simulink model "lin_att_model"  (R2024b)
settings: Solver=ode4  StartTime=0.0  StopTime=10  FixedStep=ST  RelTol=1e-3
values from neighbouring files (symbols this model uses):
  att_sp = 0    [FEL_RBFNN.m]    (also in results.m)
  B = [ 1/Ixx*lz_mr*T_mr_trim,          0,                 0 ... (first row only)    [parameters.m]
  B_inv = inv(B*B_dim)    [parameters.m]
  eta = 1    [FEL_RBFNN.m]
  f = [ 0; 0; Q_mr_trim/Izz]    [parameters.m]
  k = diag([3.7,5,10])    [FEL_RBFNN.m]
  lambda = diag([0.08,0.05,1.5])    [FEL_RBFNN.m]
  lat_cyc_range = [ -15 15 ]    [parameters.m]
  lon_cyc_range = [ -15 15 ]    [parameters.m]
  mr_coll_range = [ 7.5 25 ]    [parameters.m]
  NN_state = 1    [FEL_RBFNN.m]    (also in results.m)
  pilot_trim = [-0.11603144404 0.198191531149 -0.14266835704 0.401015389998]    [hover_trim.mat]
  sigma = linspace(1.2,4.2,neurons)'    [FEL_RBFNN.m]
  ST = 0.01    [parameters.m]
  T_flap = 16/GAMMA/OMEGA    (= 0.0932876459059)    [parameters.m]
  tr_coll_range = [ -20 20 ]    [parameters.m]
  W0 = zeros(neurons,3)    [FEL_RBFNN.m]
  x0 = linspace(-1,1,neurons)'    [FEL_RBFNN.m]
settings Model: Creator=fra62  LastModifiedBy=fra62

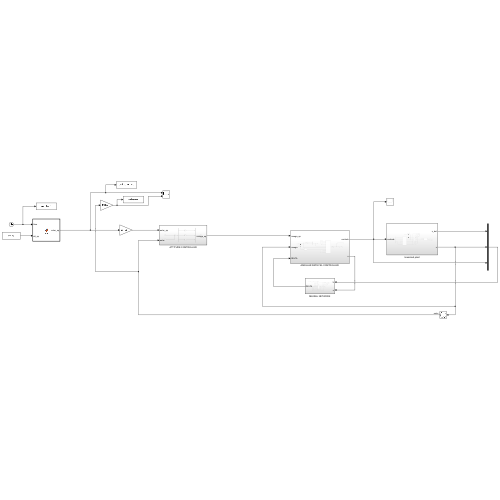
[thumbnail: Simulink's stored preview of the top-level diagram]
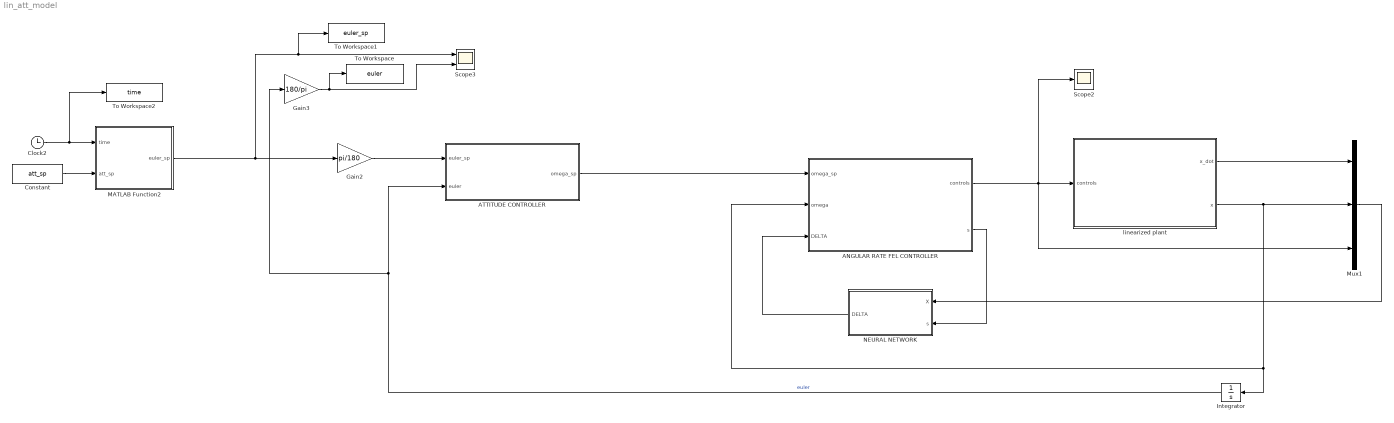
== system lin_att_model ==
  "ANGULAR RATE FEL CONTROLLER " : Subsystem
  ATTITUDE CONTROLLER : Subsystem
  Clock2 : Clock
  Constant : Constant  Value=att_sp
  Gain2 : Gain  Gain=pi/180
  Gain3 : Gain  Gain=180/pi
  Integrator : Integrator  WrapState=on
  MATLAB Function2 : MATLAB Function  TreatAsAtomicUnit=on
  Mux1 : Mux  Inputs=3
  "NEURAL NETWORK " : Subsystem
  Scope2 : Scope
  Scope3 : Scope  NumInputPorts=2
  To Workspace : ToWorkspace  VariableName=euler  SampleTime=-1
  To Workspace1 : ToWorkspace  VariableName=euler_sp  SampleTime=-1
  To Workspace2 : ToWorkspace  VariableName=time  SampleTime=-1
  linearized plant : Subsystem
  wires:
  "ANGULAR RATE FEL CONTROLLER "/1(controls) -> Scope2/1, linearized plant/1(controls), Mux1/3
  MATLAB Function2/1(euler_sp) -> Gain2/1, To Workspace1/1, Scope3/1
  Gain3/1 -> To Workspace/1, Scope3/2
  Clock2/1 -> To Workspace2/1, MATLAB Function2/1(time)
  linearized plant/2(x) -> Mux1/2, Integrator/1, "ANGULAR RATE FEL CONTROLLER "/2(omega)
  Mux1/1 -> "NEURAL NETWORK "/1(X)
  linearized plant/1(x_dot) -> Mux1/1
  "ANGULAR RATE FEL CONTROLLER "/2(s) -> "NEURAL NETWORK "/2(s)
  "NEURAL NETWORK "/1(DELTA) -> "ANGULAR RATE FEL CONTROLLER "/3(DELTA)
  Gain2/1 -> ATTITUDE CONTROLLER/1(euler_sp)
  Integrator/1 -> Gain3/1, ATTITUDE CONTROLLER/2(euler)  "euler"
  ATTITUDE CONTROLLER/1(omega_sp) -> "ANGULAR RATE FEL CONTROLLER "/1(omega_sp)
  Constant/1 -> MATLAB Function2/2(att_sp)

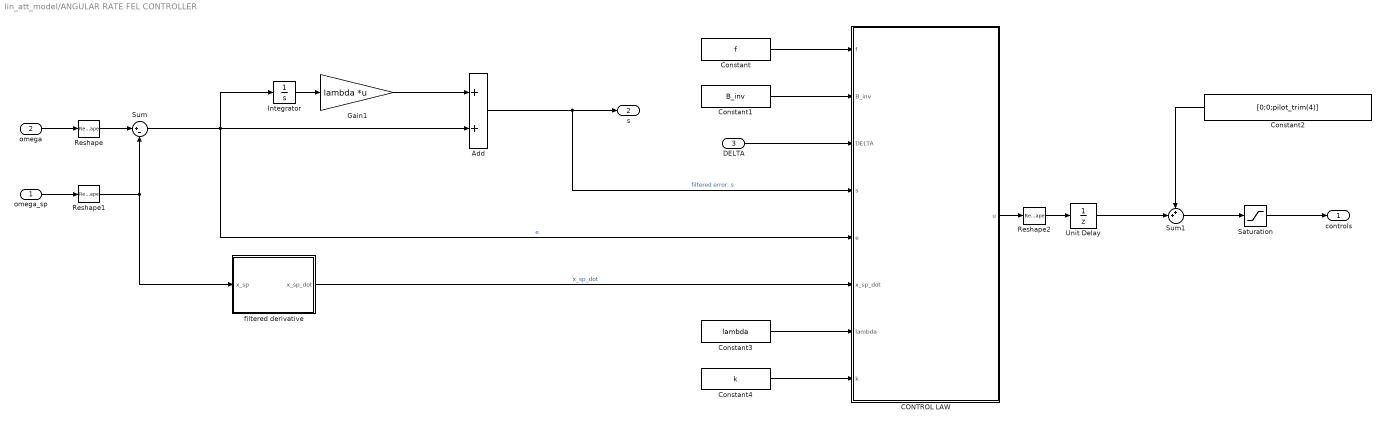
== system lin_att_model/ANGULAR RATE FEL CONTROLLER  ==
  omega_sp : Inport
  omega : Inport  Port=2
  DELTA : Inport  Port=3
  Add : Sum
  CONTROL LAW : MATLAB Function  TreatAsAtomicUnit=on
  Constant : Constant  Value=f
  Constant1 : Constant  Value=B_inv
  Constant2 : Constant  Value=[0;0;pilot_trim(4)]
  Constant3 : Constant  Value=lambda
  Constant4 : Constant  Value=k
  Gain1 : Gain  Gain=lambda  Multiplication=Matrix(K*u) (u vector)
  Integrator : Integrator
  Reshape : Reshape  OutputDimensionality=Column vector (2-D)
  Reshape1 : Reshape  OutputDimensionality=Column vector (2-D)
  Reshape2 : Reshape  OutputDimensionality=Column vector (2-D)
  Saturation : Saturate  UpperLimit=1  LowerLimit=-1
  Sum : Sum  Inputs=|+-
  Sum1 : Sum  Inputs=++|
  Unit Delay : UnitDelay  SampleTime=-1  HasFrameUpgradeWarning=on
  filtered derivative : Subsystem
  controls : Outport
  s : Outport  Port=2
  wires:
  CONTROL LAW/1(u) -> Reshape2/1
  Saturation/1 -> controls/1
  Constant/1 -> CONTROL LAW/1(f)
  Constant1/1 -> CONTROL LAW/2(B_inv)
  DELTA/1 -> CONTROL LAW/3(DELTA)
  Constant3/1 -> CONTROL LAW/7(lambda)
  Constant4/1 -> CONTROL LAW/8(k)
  omega_sp/1 -> Reshape1/1
  omega/1 -> Reshape/1
  Reshape1/1 -> filtered derivative/1(x_sp), Sum/2
  filtered derivative/1(x_sp_dot) -> CONTROL LAW/6(x_sp_dot)  "x_sp_dot"
  Sum/1 -> Integrator/1, Add/2, CONTROL LAW/5(e)  "e"
  Add/1 -> s/1, CONTROL LAW/4(s)  "filtered error: s"
  Gain1/1 -> Add/1
  Integrator/1 -> Gain1/1
  Reshape/1 -> Sum/1
  Reshape2/1 -> Unit Delay/1
  Unit Delay/1 -> Sum1/2
  Sum1/1 -> Saturation/1
  Constant2/1 -> Sum1/1

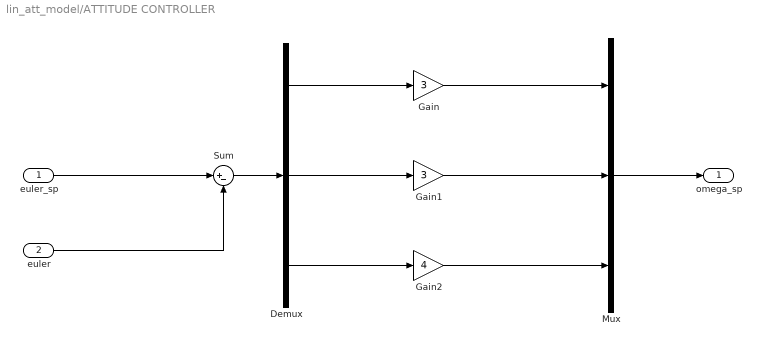
== system lin_att_model/ATTITUDE CONTROLLER ==
  euler_sp : Inport
  euler : Inport  Port=2
  Demux : Demux  Outputs=3
  Gain : Gain  Gain=3
  Gain1 : Gain  Gain=3
  Gain2 : Gain  Gain=4
  Mux : Mux  Inputs=3
  Sum : Sum  Inputs=|+-
  omega_sp : Outport
  wires:
  Gain2/1 -> Mux/3
  euler/1 -> Sum/2
  Mux/1 -> omega_sp/1
  Demux/3 -> Gain2/1
  Demux/2 -> Gain1/1
  Gain/1 -> Mux/1
  euler_sp/1 -> Sum/1
  Demux/1 -> Gain/1
  Sum/1 -> Demux/1
  Gain1/1 -> Mux/2

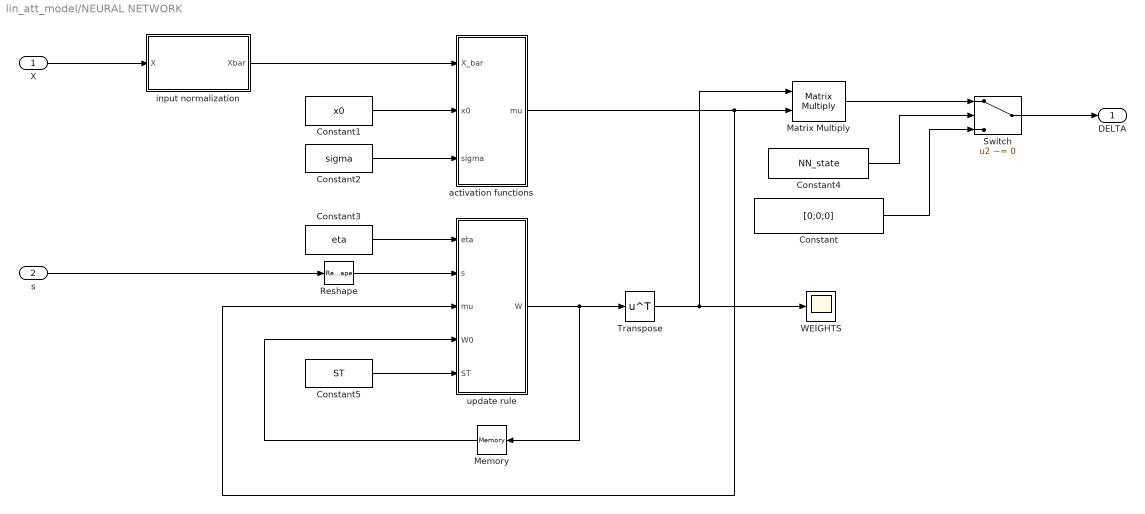
== system lin_att_model/NEURAL NETWORK  ==
  X : Inport
  s : Inport  Port=2
  Constant : Constant  Value=[0;0;0]
  Constant1 : Constant  Value=x0
  Constant2 : Constant  Value=sigma
  Constant3 : Constant  Value=eta
  Constant4 : Constant  Value=NN_state
  Constant5 : Constant  Value=ST
  Matrix Multiply : Product  Multiplication=Matrix(*)
  Memory : Memory  InitialCondition=W0
  Reshape : Reshape  OutputDimensionality=Column vector (2-D)
  Switch : Switch  Criteria=u2 ~= 0  SaturateOnIntegerOverflow=off  InputSameDT=off
  Transpose : Math  Operator=transpose
  WEIGHTS : Scope
  activation functions : MATLAB Function  TreatAsAtomicUnit=on
  input normalization : MATLAB Function  TreatAsAtomicUnit=on
  update rule : MATLAB Function  TreatAsAtomicUnit=on
  DELTA : Outport
  wires:
  Constant2/1 -> activation functions/3(sigma)
  Constant3/1 -> update rule/1(eta)
  s/1 -> Reshape/1
  X/1 -> input normalization/1(X)
  activation functions/1(mu) -> Matrix Multiply/2, update rule/3(mu)
  Constant1/1 -> activation functions/2(x0)
  input normalization/1(Xbar) -> activation functions/1(X_bar)
  Reshape/1 -> update rule/2(s)
  update rule/1(W) -> Transpose/1, Memory/1
  Transpose/1 -> Matrix Multiply/1, WEIGHTS/1
  Switch/1 -> DELTA/1
  Matrix Multiply/1 -> Switch/1
  Constant/1 -> Switch/3
  Constant4/1 -> Switch/2
  Memory/1 -> update rule/4(W0)
  Constant5/1 -> update rule/5(ST)

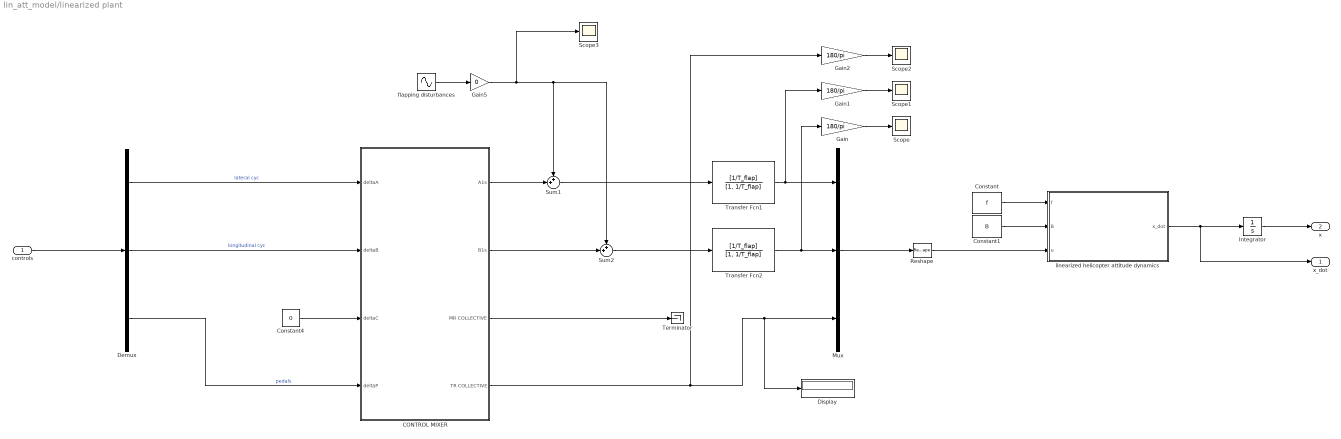
== system lin_att_model/linearized plant ==
  controls : Inport
  CONTROL MIXER : Subsystem
  Constant : Constant  Value=f
  Constant1 : Constant  Value=B
  Constant4 : Constant  Value=0
  Demux : Demux  Outputs=3
  Display : Display
  Gain : Gain  Gain=180/pi
  Gain1 : Gain  Gain=180/pi
  Gain2 : Gain  Gain=180/pi
  Gain5 : Gain  Gain=0
  Integrator : Integrator  InitialCondition=[0;0;0]
  Mux : Mux  Inputs=3
  Reshape : Reshape  OutputDimensionality=Column vector (2-D)
  Scope{,1..3} (4 alike) : Scope
  Sum1 : Sum  Inputs=++|
  Sum2 : Sum  Inputs=++|
  Terminator : Terminator
  Transfer Fcn1 : TransferFcn  Numerator=[1/T_flap]  Denominator=[1, 1/T_flap]
  Transfer Fcn2 : TransferFcn  Numerator=[1/T_flap]  Denominator=[1, 1/T_flap]
  flapping disturbances : Sin  Amplitude=0.01  Frequency=2  SampleTime=0
  linearized helicopter attitude dynamics : MATLAB Function  TreatAsAtomicUnit=on
  x_dot : Outport
  x : Outport  Port=2
  wires:
  Transfer Fcn1/1 -> Gain1/1, Mux/1
  Mux/1 -> Reshape/1
  Demux/3 -> CONTROL MIXER/4(deltaP)  "pedals"
  CONTROL MIXER/4(TR COLLECTIVE) -> Gain2/1, Display/1, Mux/3
  Constant4/1 -> CONTROL MIXER/3(deltaC)
  Transfer Fcn2/1 -> Gain/1, Mux/2
  Demux/2 -> CONTROL MIXER/2(deltaB)  "longitudinal cyc"
  CONTROL MIXER/3(MR COLLECTIVE) -> Terminator/1
  Demux/1 -> CONTROL MIXER/1(deltaA)  "lateral cyc"
  controls/1 -> Demux/1
  Gain/1 -> Scope/1
  Gain1/1 -> Scope1/1
  Gain2/1 -> Scope2/1
  Constant/1 -> linearized helicopter attitude dynamics/1(f)
  Constant1/1 -> linearized helicopter attitude dynamics/2(B)
  linearized helicopter attitude dynamics/1(x_dot) -> x_dot/1, Integrator/1
  Reshape/1 -> linearized helicopter attitude dynamics/3(u)
  CONTROL MIXER/1(A1s) -> Sum1/2
  Sum1/1 -> Transfer Fcn1/1
  CONTROL MIXER/2(B1s) -> Sum2/2
  Sum2/1 -> Transfer Fcn2/1
  flapping disturbances/1 -> Gain5/1
  Gain5/1 -> Scope3/1, Sum1/1, Sum2/1
  Integrator/1 -> x/1

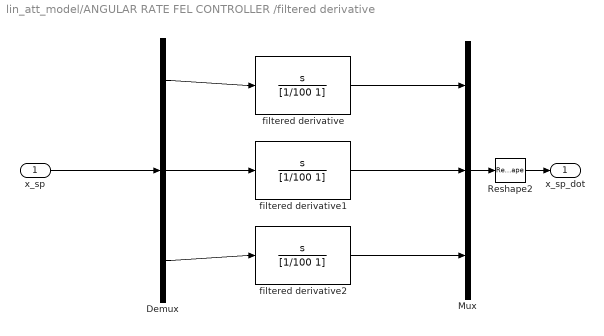
== system lin_att_model/ANGULAR RATE FEL CONTROLLER /filtered derivative ==
  x_sp : Inport
  Demux : Demux  Outputs=3
  Mux : Mux  Inputs=3
  Reshape2 : Reshape  OutputDimensionality=Column vector (2-D)
  filtered derivative : TransferFcn  Numerator=[1 0]  Denominator=[1/100 1]
  filtered derivative1 : TransferFcn  Numerator=[1 0]  Denominator=[1/100 1]
  filtered derivative2 : TransferFcn  Numerator=[1 0]  Denominator=[1/100 1]
  x_sp_dot : Outport
  wires:
  Demux/3 -> filtered derivative2/1
  Demux/1 -> filtered derivative/1
  Mux/1 -> Reshape2/1
  Demux/2 -> filtered derivative1/1
  filtered derivative1/1 -> Mux/2
  x_sp/1 -> Demux/1
  filtered derivative/1 -> Mux/1
  filtered derivative2/1 -> Mux/3
  Reshape2/1 -> x_sp_dot/1

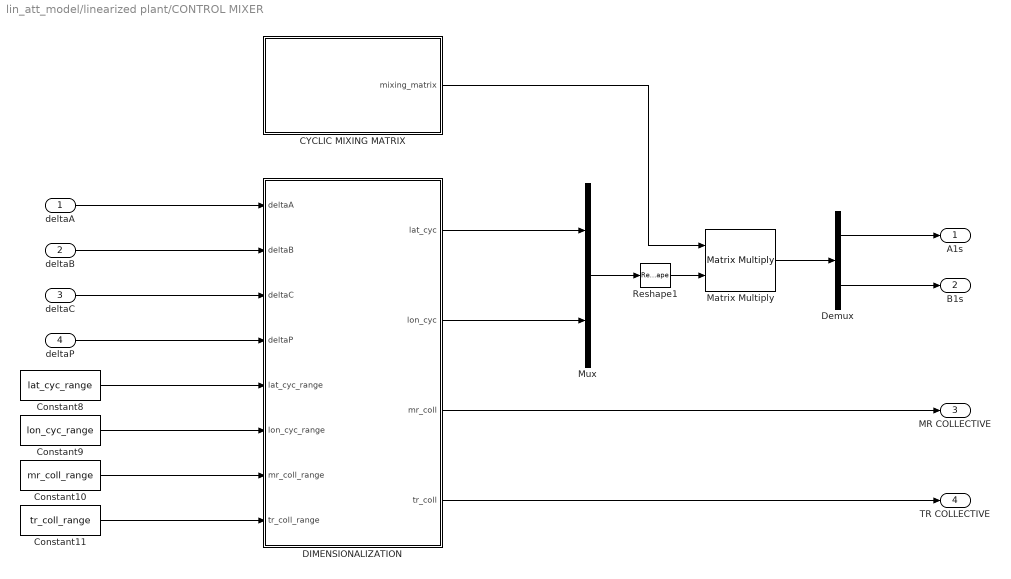
== system lin_att_model/linearized plant/CONTROL MIXER ==
  deltaA : Inport
  deltaB : Inport  Port=2
  deltaC : Inport  Port=3
  deltaP : Inport  Port=4
  CYCLIC MIXING MATRIX : MATLAB Function  TreatAsAtomicUnit=on
  Constant10 : Constant  Value=mr_coll_range
  Constant11 : Constant  Value=tr_coll_range
  Constant8 : Constant  Value=lat_cyc_range
  Constant9 : Constant  Value=lon_cyc_range
  DIMENSIONALIZATION : MATLAB Function  TreatAsAtomicUnit=on
  Demux : Demux  Outputs=2
  Matrix Multiply : Product  Multiplication=Matrix(*)
  Mux : Mux  Inputs=2
  Reshape1 : Reshape  OutputDimensionality=Column vector (2-D)
  A1s : Outport
  B1s : Outport  Port=2
  MR COLLECTIVE : Outport  Port=3
  TR COLLECTIVE : Outport  Port=4
  wires:
  Demux/2 -> B1s/1
  Matrix Multiply/1 -> Demux/1
  Mux/1 -> Reshape1/1
  Demux/1 -> A1s/1
  CYCLIC MIXING MATRIX/1(mixing_matrix) -> Matrix Multiply/1
  DIMENSIONALIZATION/1(lat_cyc) -> Mux/1
  DIMENSIONALIZATION/2(lon_cyc) -> Mux/2
  deltaP/1 -> DIMENSIONALIZATION/4(deltaP)
  deltaC/1 -> DIMENSIONALIZATION/3(deltaC)
  deltaB/1 -> DIMENSIONALIZATION/2(deltaB)
  deltaA/1 -> DIMENSIONALIZATION/1(deltaA)
  DIMENSIONALIZATION/3(mr_coll) -> MR COLLECTIVE/1
  DIMENSIONALIZATION/4(tr_coll) -> TR COLLECTIVE/1
  Constant8/1 -> DIMENSIONALIZATION/5(lat_cyc_range)
  Constant9/1 -> DIMENSIONALIZATION/6(lon_cyc_range)
  Constant10/1 -> DIMENSIONALIZATION/7(mr_coll_range)
  Constant11/1 -> DIMENSIONALIZATION/8(tr_coll_range)
  Reshape1/1 -> Matrix Multiply/2

== matlab function lin_att_model/ANGULAR RATE FEL CONTROLLER /CONTROL LAW ==
  data: f input; u output; B_inv input; DELTA input; s input; e input; x_sp_dot input; lambda input; k input
function u = fcn(f,B_inv,DELTA,s,e,x_sp_dot,lambda,k)


u = B_inv*(-f-DELTA+x_sp_dot-lambda*e-k*s);

== matlab function lin_att_model/MATLAB Function2 ==
  data: time input; euler_sp output; att_sp input
function euler_sp = fcn(time,att_sp)

T = 15;

if att_sp == 2
    phi_sp   = 10*cos(2*pi*time/T-pi/3);
    theta_sp = 5*cos(2*pi*time/T-pi/3);
    psi_sp   = 10*cos(2*pi*time/T-pi/3);
elseif att_sp == 1
    phi_sp   = 10;
    theta_sp = 5;
    psi_sp   = 15;
else
    phi_sp   = 0;
    theta_sp = 0;
    psi_sp   = 0;
end

euler_sp = [phi_sp;theta_sp;psi_sp];

== matlab function lin_att_model/NEURAL NETWORK /activation functions ==
  data: X_bar input; x0 input; sigma input; mu output
function mu = fcn(X_bar, x0, sigma)

mu = x0*0;
for i=1:length(mu)
    mu(i,1) = exp(-((X_bar-x0(i))'*(X_bar-x0(i)))/(2*sigma(i)^2));
end

== matlab function lin_att_model/NEURAL NETWORK /input normalization ==
  data: X input; Xbar output
function Xbar = fcn(X)

% X = [ phidot,thetadot,psidot, phi,theta,psi, deltaA,deltaB,deltaP ]
% controls are already normalized

max_rate  = 2;      % expected max angular rate [rad/s]
max_angle = pi/2;   % expected max attitude angle [rad]

Xbar = [  X(1)/max_rate ;
          X(2)/max_rate ;
          X(3)/max_rate ;
          X(4)/max_angle;
          X(5)/max_angle;
          X(6)/max_angle;
          X(7)          ;
          X(8)          ;
          X(9)          ];

== matlab function lin_att_model/NEURAL NETWORK /update rule ==
  data: eta input; s input; mu input; W output; W0 input; ST input
function W = fcn(eta,s,mu,W0,ST)

sigma = 0.01;
dWdt = eta*(mu*s'-sigma*W0);
W = W0+dWdt*ST;

== matlab function lin_att_model/linearized plant/CONTROL MIXER/CYCLIC MIXING MATRIX ==
  data: mixing_matrix output
function mixing_matrix = fcn()

mixing_matrix = [1  0;
                 0 -1];

== matlab function lin_att_model/linearized plant/CONTROL MIXER/DIMENSIONALIZATION ==
  data: deltaA input; deltaB input; deltaC input; deltaP input; lat_cyc output; lon_cyc output; mr_coll output; tr_coll output; lat_cyc_range input; lon_cyc_range input; mr_coll_range input; tr_coll_range input
function [lat_cyc,lon_cyc,mr_coll,tr_coll] = fcn(deltaA,deltaB,deltaC,deltaP,lat_cyc_range,lon_cyc_range,mr_coll_range,tr_coll_range)

lat_cyc = (deltaA*0.5*(lat_cyc_range(2)-lat_cyc_range(1))+0.5*(lat_cyc_range(2)+lat_cyc_range(1)))*pi/180;
lon_cyc = (deltaB*0.5*(lon_cyc_range(2)-lon_cyc_range(1))+0.5*(lon_cyc_range(2)+lon_cyc_range(1)))*pi/180;
mr_coll = (deltaC*0.5*(mr_coll_range(2)-mr_coll_range(1))+0.5*(mr_coll_range(2)+mr_coll_range(1)))*pi/180;
tr_coll = (deltaP*0.5*(tr_coll_range(2)-tr_coll_range(1))+0.5*(tr_coll_range(2)+tr_coll_range(1)))*pi/180;

== matlab function lin_att_model/linearized plant/linearized helicopter attitude dynamics ==
  data: f input; B input; u input; x_dot output
function x_dot = fcn(f,B,u)

x_dot = f + B*u;
